simulink model "mck2"  (R2022a)
settings: Solver=VariableStepAuto  StartTime=0.0  StopTime=10.0  RelTol=1e-3
PreLoadFcn:
  | m=0.1;
  | c=0.2;
  | k=0.5;
  | F=10;
settings Model: Creator=seong  LastModifiedBy=pc
settings SolverCC: AlgebraicLoopSolver=TrustRegion
settings DataIOCC: SaveFormat=Array  OutputSaveName=xout
settings DebuggingCC: UnconnectedInputMsg=warning  UnconnectedOutputMsg=warning  UnconnectedLineMsg=warning  SFMachineParentedDataDiag=warning
settings SFSimCC: CustomCodeUndefinedFunction=UseInterfaceOnly

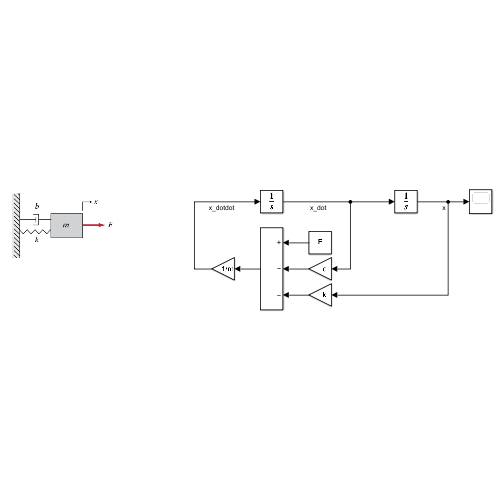
[thumbnail: Simulink's stored preview of the top-level diagram]
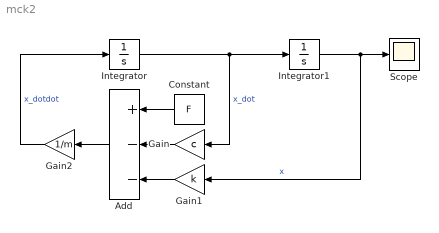
== system mck2 ==
  Add : Sum  Inputs=+--
  Constant : Constant  Value=F
  Gain : Gain  Gain=c
  Gain1 : Gain  Gain=k
  Gain2 : Gain  Gain=1/m
  Integrator : Integrator  InitialCondition=10
  Integrator1 : Integrator
  Scope : Scope
  wires:
  Integrator/1 -> Gain/1, Integrator1/1  "x_dot"
  Gain2/1 -> Integrator/1  "x_dotdot"
  Integrator1/1 -> Scope/1, Gain1/1  "x"
  Gain/1 -> Add/2
  Gain1/1 -> Add/3
  Add/1 -> Gain2/1
  Constant/1 -> Add/1
